simulink model "house_model1_onoff"  (Simulink 7.6)
settings: Solver=ode45  StartTime=0.0  StopTime=4*3600  RelTol=1e-3
values from neighbouring files (symbols this model uses):
  C_R = 100000    [Simulation.m]
  H = 2    [Simulation.m]
  K = 100    [Simulation.m]
  Q_F_ON = 1000    [Simulation.m]
  Q_H = 1500    [Simulation.m]
  t_a = 0    [Simulation.m]
  t_init = 5    [Simulation.m]
  t_R_set = 20    [Simulation.m]
  tau_F = 2*3600    (= 7200)    [Simulation.m]
  tau_s = 60    [Simulation.m]
libraries: simulink_extras x1
settings Model: Creator=sgt  LastModifiedBy=sgt
settings OptimizationCC: InlineInvariantSignals=on  InitFltsAndDblsToZero=on
settings DebuggingCC: SaveWithParameterizedLinksMsg=none  SignalResolutionControl=TryResolveAllWithWarning  MultiTaskDSMMsg=warning  MultiTaskCondExecSysMsg=none  StrictBusMsg=None
settings RTWCC: IncludeERTFirstTime=on
settings GRTTargetCC: TargetFcnLib=ansi_tfl_tmw.mat

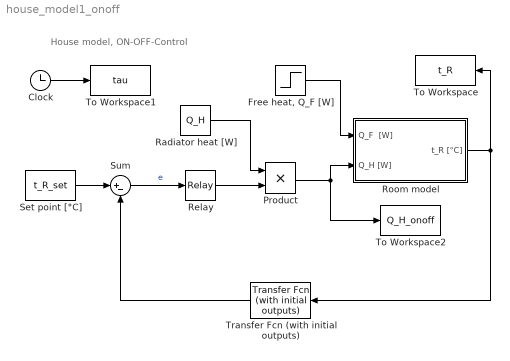
== system house_model1_onoff ==
  note: House model, ON-OFF-Control
  Clock : Clock
      settings: Decimation=10
  "Free heat, Q_F [W]" : Step  Time=tau_F  After=Q_F_ON  SampleTime=0
  Product : Product  RndMeth=Zero
  Radiator heat [W] : Constant  Value=Q_H
  Relay : Relay  OnSwitchValue=H/2  OffSwitchValue=-H/2
  Room model : Subsystem
  Set point [°C] : Constant  Value=t_R_set
  Sum : Sum  Inputs=|+-
  To Workspace : ToWorkspace  VariableName=t_R  SampleTime=-1  SaveFormat=Array
  To Workspace1 : ToWorkspace  VariableName=tau  SampleTime=-1  SaveFormat=Array
  To Workspace2 : ToWorkspace  VariableName=Q_H_onoff  SampleTime=-1  SaveFormat=Array
  Transfer Fcn (with initial outputs) : simulink_extras/Additional Linear/Transfer Fcn (with initial outputs)  SystemSampleTime=-1  N=[1]  D="[tau_s  1]"  Y0=t_init  U0=0
  wires:
  Clock/1 -> To Workspace1/1
  "Free heat, Q_F [W]"/1 -> Room model/1(Q_F  [W])
  Room model/1(t_R [°C]) -> To Workspace/1, Transfer Fcn (with initial outputs)/1
  Product/1 -> Room model/2(Q_H [W]), To Workspace2/1
  Relay/1 -> Product/2
  Radiator heat [W]/1 -> Product/1
  Set point [°C]/1 -> Sum/1
  Transfer Fcn (with initial outputs)/1 -> Sum/2
  Sum/1 -> Relay/1  "e"

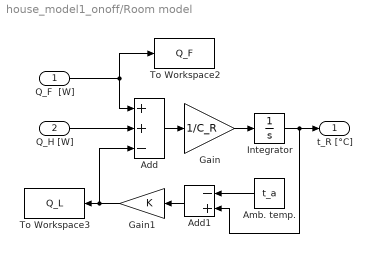
== system house_model1_onoff/Room model ==
  Q_F  [W] : Inport
  Q_H [W] : Inport  Port=2
  Add : Sum  Inputs=++-
  Add1 : Sum  Inputs=-+
  Amb. temp. : Constant  Value=t_a
  Gain : Gain  Gain=1/C_R
  Gain1 : Gain  Gain=K
  Integrator : Integrator  InitialCondition=t_init
  To Workspace2 : ToWorkspace  VariableName=Q_F  SampleTime=-1  SaveFormat=Array
  To Workspace3 : ToWorkspace  VariableName=Q_L  SampleTime=-1  SaveFormat=Array
  t_R [°C] : Outport
  wires:
  Integrator/1 -> Add1/2, t_R [°C]/1
  Gain/1 -> Integrator/1
  Add/1 -> Gain/1
  Q_F  [W]/1 -> To Workspace2/1, Add/1
  Amb. temp./1 -> Add1/1
  Add1/1 -> Gain1/1
  Gain1/1 -> Add/3, To Workspace3/1
  Q_H [W]/1 -> Add/2
